simulink model "test_hill_sim"  (R2014b)
settings: Solver=ode113  StartTime=0.0  StopTime=t_end_CW  MaxStep=1e-3  MinStep=1e-12  RelTol=1e-9  AbsTol=1e-4
values from neighbouring files (symbols this model uses):
  a_sat = f_sat/m_cubesat    (= 0.0004)    [Controlled_motion_test1.m]    (also in Hill_TEST.m; TRAJ_Hill_test.m; controlled_motion_test2.m = 0.001)
  h_orb = 400*10^3    (= 400000)    [ATV_laplace_potentials_test0.m]    (also in CW_anlytical.m = 200000; Controlled_motion_test1.m; EOS_test.m = 250000; Hill_TEST.m = 800000)
  K_lqr = -K    [Controlled_motion_test1.m]    (also in Hill_TEST.m; TRAJ_Hill_test.m; controlled_motion_test2.m)
  Kp = kp    (= -0.075)    [Controlled_motion_test1.m]    (also in Hill_TEST.m = -7.5e-05; controlled_motion_test2.m; r2BP_t_c_CTR_SP.m = [kp 0 0)
  Kv = kv    (= -50)    [Controlled_motion_test1.m]    (also in Hill_TEST.m = -0.05; controlled_motion_test2.m; r2BP_t_c_CTR_SP.m = [kv 0 0)
  m_cubesat = 5    [Controlled_motion_test1.m]    (also in Hill_TEST.m; TRAJ_Hill_test.m; controlled_motion_test2.m)
  Mu = (3.9856e+14)    (= 398560000000000)    [ATV_laplace_potentials_test0.m]    (also in CW_anlytical.m; Controlled_motion_test1.m; EOS_test.m; Hill_TEST.m)
  R_0c = (R_0t+rand(3,1)*0.25*1e2)    [ATV_laplace_potentials_test0.m]    (also in CW_anlytical.m = [R_C;0;0]; Controlled_motion_test1.m = (R_0t+X_obs+rand(3,1)*0.25*1e2); Hill_TEST.m = (R_0t-rand(3,1)*0.5*1e2); Hill_TEST_INTEGR.m = (R_0t-[d_TC;0;0]))
  R_0t = [R_T;0;0]    [CW_anlytical.m]    (also in Controlled_motion_test1.m = [(r_Earth+h_orb);0;0]; EOS_test.m = [(r_Earth+h_orb);0;0]; Hill_TEST.m = [(r_Earth+h_orb);0;0]; Hill_TEST_INTEGR.m = [(r_Earth+h_orb);0;0])
  V_0c = (V_0t+rand(3,1)*0.5*1e-1)    [ATV_laplace_potentials_test0.m]    (also in CW_anlytical.m = [0;sqrt(Mu/norm(R_0c));0]; Controlled_motion_test1.m = (V_0t-rand(3,1)*0.25*1e-2); Hill_TEST.m; Hill_TEST_INTEGR.m = [0;omega*R_C;0])
  V_0t = [0;sqrt(Mu/(r_Earth+h_orb));0]    [CW_anlytical.m]    (also in Controlled_motion_test1.m; EOS_test.m; Hill_TEST.m; Hill_TEST_INTEGR.m)
undefined symbols (not defined in the file or in its folder): E, E_Moon, r_0, v_0
libraries: dspmtrx3 x4, vrlib x2
settings Model: Creator=peace  LastModifiedBy=peace

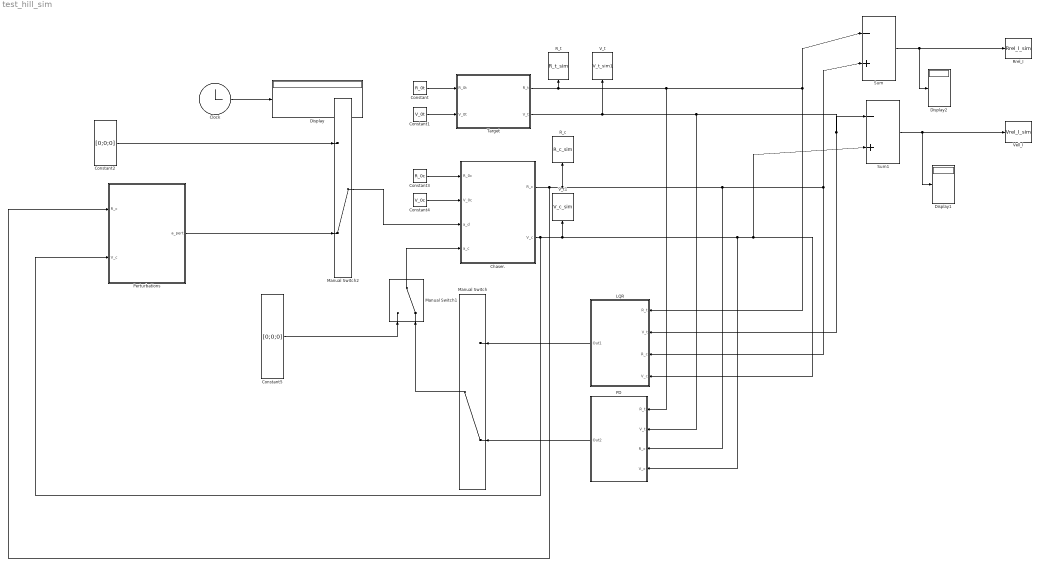
== system test_hill_sim ==
  Chaser. : Subsystem
  Clock : Clock
  Constant : Constant  Value=R_0t  VectorParams1D=off
  Constant1 : Constant  Value=V_0t  VectorParams1D=off
  Constant2 : Constant  Value=[0;0;0]  VectorParams1D=off
  Constant3 : Constant  Value=R_0c  VectorParams1D=off
  Constant4 : Constant  Value=V_0c  VectorParams1D=off
  Constant5 : Constant  Value=[0;0;0]  VectorParams1D=off
  Display : Display
  Display1 : Display
  Display2 : Display
  LQR : Subsystem
  Manual Switch : ManualSwitch  CurrentSetting=0
  Manual Switch1 : ManualSwitch  CurrentSetting=0
  Manual Switch2 : ManualSwitch  CurrentSetting=0
  PD : Subsystem
  Perturbations : Subsystem
  R_c : ToWorkspace  VariableName=R_c_sim  SaveFormat=Structure With Time  SampleTime=-1
  R_t : ToWorkspace  VariableName=R_t_sim  SaveFormat=Structure With Time  SampleTime=-1
  Rrel_I : ToWorkspace  VariableName=Rrel_I_sim  SaveFormat=Structure With Time  SampleTime=-1
  Sum : Sum  Inputs=|-+
  Sum1 : Sum  Inputs=|-+
  Target : Subsystem
  V_t : ToWorkspace  VariableName=V_t_sim1  SaveFormat=Structure With Time  SampleTime=-1
  V_t1 : ToWorkspace  VariableName=V_c_sim  SaveFormat=Structure With Time  SampleTime=-1
  Vell_I : ToWorkspace  VariableName=Vrel_I_sim  SaveFormat=Structure With Time  SampleTime=-1
  wires:
  Target/1(R_t) -> R_t/1, PD/1(R_t), LQR/1(R_t), Sum/1
  Constant/1 -> Target/1(R_0t)
  Constant1/1 -> Target/2(V_0t)
  Constant3/1 -> Chaser./1(R_0c)
  Constant4/1 -> Chaser./2(V_0c)
  Target/2("V_t ") -> V_t/1, PD/2(V_t), Sum1/1, LQR/2(V_t)
  Chaser./1(R_c) -> PD/3(R_c), LQR/3(R_c), Sum/2, R_c/1, Perturbations/1("R_c ")
  Chaser./2(V_c) -> Perturbations/2("V_c "), Sum1/2, LQR/4(V_c), PD/4(V_c), V_t1/1
  LQR/1(Out1) -> Manual Switch/1
  PD/1(Out2) -> Manual Switch/2
  Manual Switch1/1 -> Chaser./4(a_c)
  Constant5/1 -> Manual Switch1/1
  Manual Switch/1 -> Manual Switch1/2
  Perturbations/1(a_pert) -> Manual Switch2/2
  Manual Switch2/1 -> Chaser./3(a_d)
  Constant2/1 -> Manual Switch2/1
  Clock/1 -> Display/1
  Sum/1 -> Display2/1, Rrel_I/1
  Sum1/1 -> Display1/1, Vell_I/1

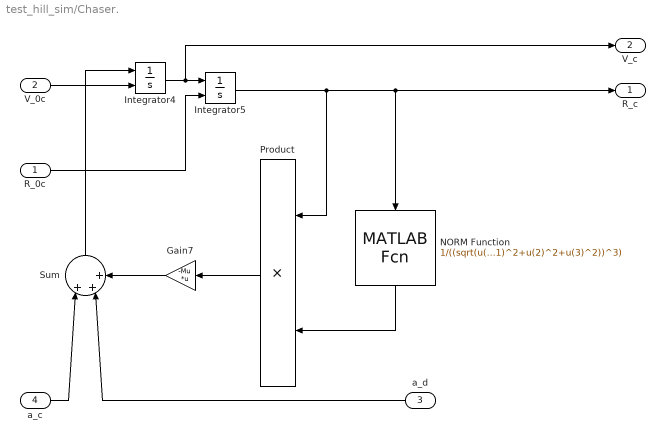
== system test_hill_sim/Chaser. ==
  R_0c : Inport
  V_0c : Inport  Port=2
  a_d : Inport  Port=3
  a_c : Inport  Port=4
  Gain7 : Gain  Gain=-Mu  Multiplication=Matrix(K*u)
  Integrator4 : Integrator  InitialConditionSource=external  InitialCondition=v_0
  Integrator5 : Integrator  InitialConditionSource=external  InitialCondition=r_0
  NORM Function : MATLABFcn  MATLABFcn=1/((sqrt(u(1)^2+u(2)^2+u(3)^2))^3)  OutputDimensions=1
  Product : Product
  Sum : Sum  Inputs=|+++
  R_c : Outport
  V_c : Outport  Port=2
  wires:
  Integrator5/1 -> R_c/1, NORM Function/1, Product/1
  Integrator4/1 -> Integrator5/1, V_c/1
  Product/1 -> Gain7/1
  NORM Function/1 -> Product/2
  V_0c/1 -> Integrator4/2
  R_0c/1 -> Integrator5/2
  Gain7/1 -> Sum/3
  Sum/1 -> Integrator4/1
  a_d/1 -> Sum/2
  a_c/1 -> Sum/1

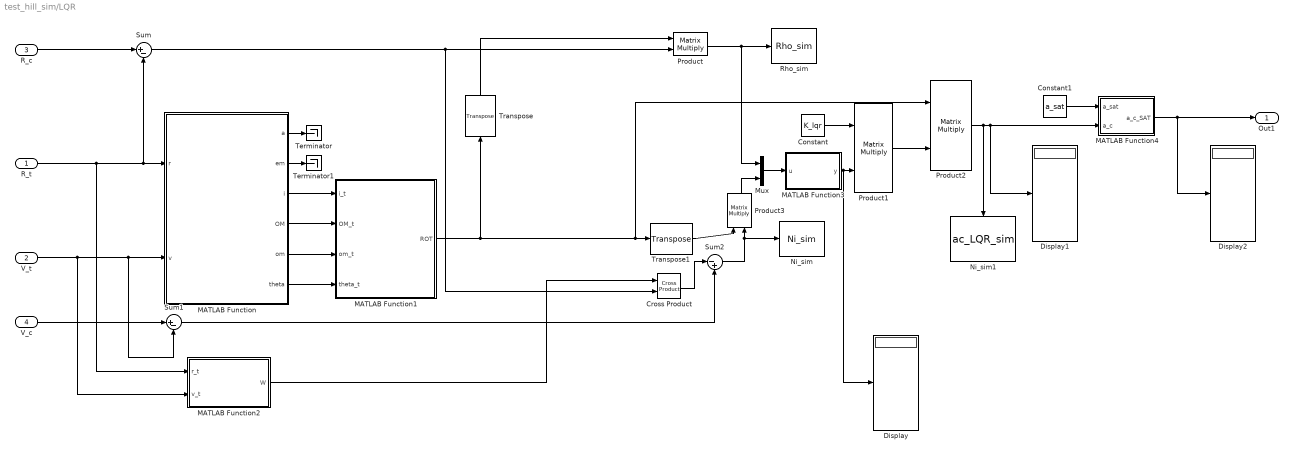
== system test_hill_sim/LQR ==
  R_t : Inport
  V_t : Inport  Port=2
  R_c : Inport  Port=3
  V_c : Inport  Port=4
  Constant : Constant  Value=K_lqr  VectorParams1D=off
  Constant1 : Constant  Value=a_sat
  Cross Product : vrlib/Utilities/Cross Product
  Display : Display
  Display1 : Display
  Display2 : Display
  MATLAB Function : MATLAB Function  TreatAsAtomicUnit=on
  MATLAB Function1 : MATLAB Function  TreatAsAtomicUnit=on
  MATLAB Function2 : MATLAB Function  TreatAsAtomicUnit=on
  MATLAB Function3 : MATLAB Function  TreatAsAtomicUnit=on
  MATLAB Function4 : MATLAB Function  TreatAsAtomicUnit=on
  Mux : Mux  Inputs=2
  Ni_sim : ToWorkspace  VariableName=Ni_sim  SaveFormat=Structure With Time  SampleTime=-1
  Ni_sim1 : ToWorkspace  VariableName=ac_LQR_sim  SaveFormat=Structure With Time  SampleTime=-1
  Product{,1..3} (4 alike) : Product  Multiplication=Matrix(*)
  Rho_sim : ToWorkspace  VariableName=Rho_sim  SaveFormat=Structure With Time  SampleTime=-1
  Sum : Sum  Inputs=|+-
  Sum1 : Sum  Inputs=|+-
  Sum2 : Sum  Inputs=|-+
  Terminator : Terminator
  Terminator1 : Terminator
  Transpose : dspmtrx3/Transpose  Hermitian=off  overflowFlag=off
  Transpose1 : dspmtrx3/Transpose  Hermitian=off  overflowFlag=off
  Out1 : Outport
  wires:
  R_t/1 -> Sum/2, MATLAB Function/1(r), MATLAB Function2/1(r_t)
  V_t/1 -> Sum1/2, MATLAB Function/2(v), MATLAB Function2/2(v_t)
  MATLAB Function/1(a) -> Terminator/1
  MATLAB Function/2(em) -> Terminator1/1
  MATLAB Function/3(i) -> MATLAB Function1/1(i_t)
  MATLAB Function/6(theta) -> MATLAB Function1/4(theta_t)
  MATLAB Function/4(OM) -> MATLAB Function1/2(OM_t)
  MATLAB Function/5(om) -> MATLAB Function1/3(om_t)
  R_c/1 -> Sum/1
  MATLAB Function1/1(ROT) -> Transpose/1, Product2/1, Transpose1/1
  V_c/1 -> Sum1/1
  Sum1/1 -> Sum2/2
  Sum/1 -> Product/2, Cross Product/2
  Cross Product/1 -> Sum2/1
  Product/1 -> Mux/1, Rho_sim/1
  Sum2/1 -> Product3/2, Ni_sim/1
  Constant/1 -> Product1/1
  Product2/1 -> MATLAB Function4/2(a_c), Display1/1, Ni_sim1/1
  Product1/1 -> Product2/2
  MATLAB Function2/1(W) -> Cross Product/1
  Transpose/1 -> Product/1
  Transpose1/1 -> Product3/1
  Product3/1 -> Mux/2
  Mux/1 -> MATLAB Function3/1(u)
  MATLAB Function3/1(y) -> Display/1, Product1/2
  MATLAB Function4/1(a_c_SAT) -> Display2/1, Out1/1
  Constant1/1 -> MATLAB Function4/1(a_sat)

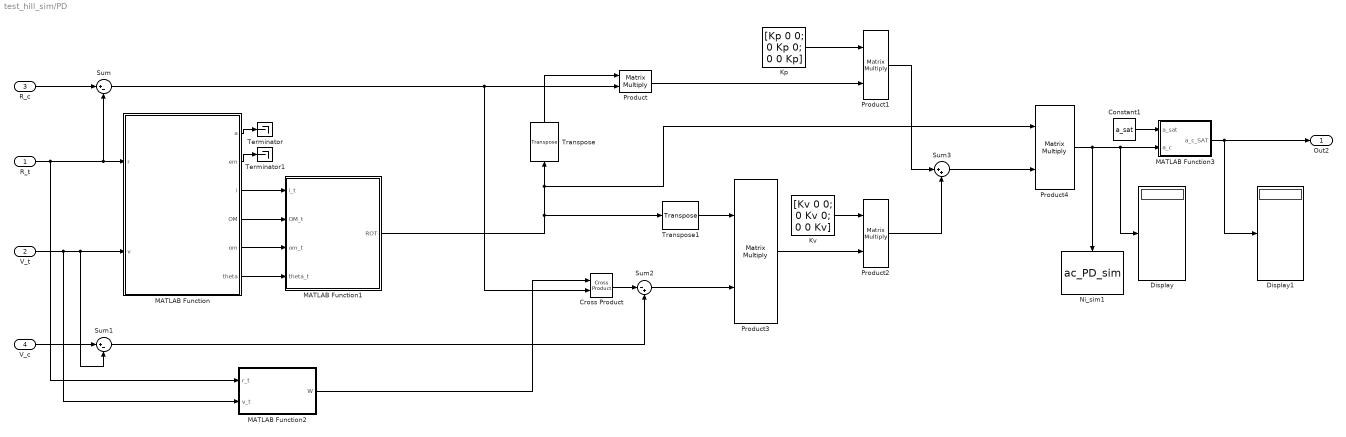
== system test_hill_sim/PD ==
  R_t : Inport
  V_t : Inport  Port=2
  R_c : Inport  Port=3
  V_c : Inport  Port=4
  Constant1 : Constant  Value=a_sat
  Cross Product : vrlib/Utilities/Cross Product
  Display : Display
  Display1 : Display
  Kp : Constant  Value=[Kp 0 0; 0 Kp 0; 0 0 Kp]  VectorParams1D=off
  Kv : Constant  Value=[Kv 0 0; 0 Kv 0; 0 0 Kv]  VectorParams1D=off
  MATLAB Function : MATLAB Function  TreatAsAtomicUnit=on
  MATLAB Function1 : MATLAB Function  TreatAsAtomicUnit=on
  MATLAB Function2 : MATLAB Function  TreatAsAtomicUnit=on
  MATLAB Function3 : MATLAB Function  TreatAsAtomicUnit=on
  Ni_sim1 : ToWorkspace  VariableName=ac_PD_sim  SaveFormat=Structure With Time  SampleTime=-1
  Product{,1..4} (5 alike) : Product  Multiplication=Matrix(*)
  Sum : Sum  Inputs=|+-
  Sum1 : Sum  Inputs=|+-
  Sum2 : Sum  Inputs=|-+
  Sum3 : Sum  Inputs=|++
  Terminator : Terminator
  Terminator1 : Terminator
  Transpose : dspmtrx3/Transpose  Hermitian=off  overflowFlag=off
  Transpose1 : dspmtrx3/Transpose  Hermitian=off  overflowFlag=off
  Out2 : Outport
  wires:
  R_t/1 -> MATLAB Function/1(r), Sum/2, MATLAB Function2/1(r_t)
  V_t/1 -> MATLAB Function2/2(v_t), MATLAB Function/2(v), Sum1/2
  MATLAB Function/1(a) -> Terminator/1
  MATLAB Function/2(em) -> Terminator1/1
  MATLAB Function/3(i) -> MATLAB Function1/1(i_t)
  MATLAB Function/6(theta) -> MATLAB Function1/4(theta_t)
  MATLAB Function/4(OM) -> MATLAB Function1/2(OM_t)
  MATLAB Function/5(om) -> MATLAB Function1/3(om_t)
  R_c/1 -> Sum/1
  MATLAB Function1/1(ROT) -> Product4/1, Transpose/1, Transpose1/1
  V_c/1 -> Sum1/1
  Sum1/1 -> Sum2/2
  Cross Product/1 -> Sum2/1
  Product/1 -> Product1/2
  Kp/1 -> Product1/1
  Kv/1 -> Product2/1
  Sum2/1 -> Product3/2
  Product3/1 -> Product2/2
  Product2/1 -> Sum3/2
  Product1/1 -> Sum3/1
  Product4/1 -> Ni_sim1/1, MATLAB Function3/2(a_c), Display/1
  Sum3/1 -> Product4/2
  Sum/1 -> Product/2, Cross Product/2
  Transpose/1 -> Product/1
  MATLAB Function2/1(W) -> Cross Product/1
  Transpose1/1 -> Product3/1
  Constant1/1 -> MATLAB Function3/1(a_sat)
  MATLAB Function3/1(a_c_SAT) -> Display1/1, Out2/1

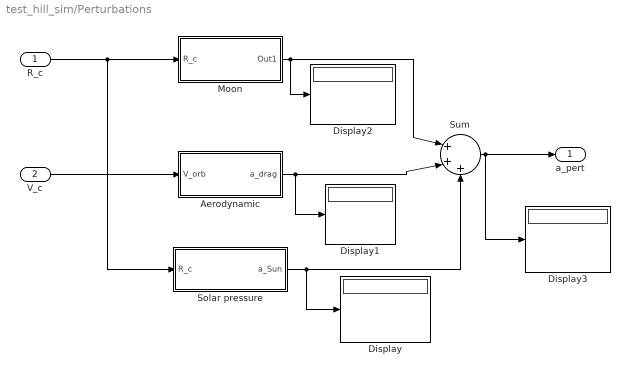
== system test_hill_sim/Perturbations ==
  "R_c " : Inport
  "V_c " : Inport  Port=2
  Aerodynamic : Subsystem
  Display{,1..3} (4 alike) : Display
  Moon : Subsystem
  Solar pressure : Subsystem
  Sum : Sum  Inputs=|+++
  a_pert : Outport
  wires:
  "R_c "/1 -> Solar pressure/1(R_c), Moon/1(R_c)
  Moon/1(Out1) -> Display2/1, Sum/1
  Sum/1 -> Display3/1, a_pert/1
  Aerodynamic/1(a_drag) -> Display1/1, Sum/2
  Solar pressure/1("a_Sun ") -> Display/1, Sum/3
  "V_c "/1 -> Aerodynamic/1(V_orb)

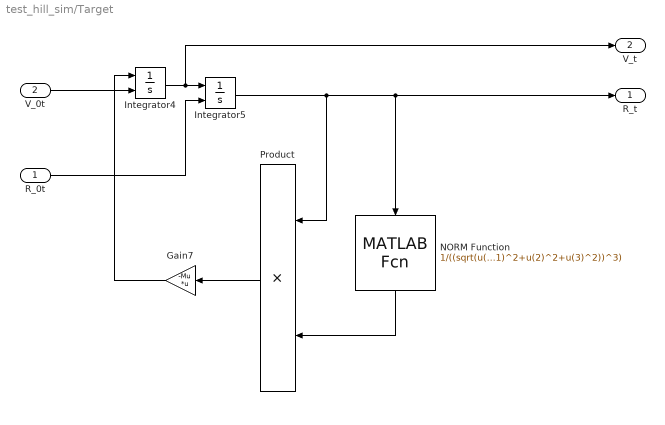
== system test_hill_sim/Target ==
  R_0t : Inport
  V_0t : Inport  Port=2
  Gain7 : Gain  Gain=-Mu  Multiplication=Matrix(K*u)
  Integrator4 : Integrator  InitialConditionSource=external  InitialCondition=v_0
  Integrator5 : Integrator  InitialConditionSource=external  InitialCondition=r_0
  NORM Function : MATLABFcn  MATLABFcn=1/((sqrt(u(1)^2+u(2)^2+u(3)^2))^3)  OutputDimensions=1
  Product : Product
  R_t : Outport
  "V_t " : Outport  Port=2
  wires:
  Integrator5/1 -> R_t/1, NORM Function/1, Product/1
  Integrator4/1 -> Integrator5/1, "V_t "/1
  Gain7/1 -> Integrator4/1
  Product/1 -> Gain7/1
  NORM Function/1 -> Product/2
  V_0t/1 -> Integrator4/2
  R_0t/1 -> Integrator5/2

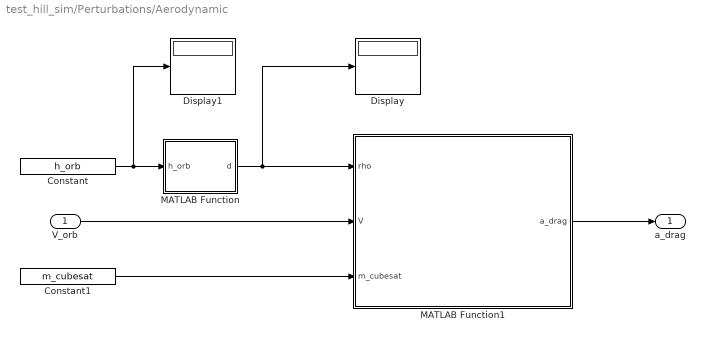
== system test_hill_sim/Perturbations/Aerodynamic ==
  V_orb : Inport
  Constant : Constant  Value=h_orb
  Constant1 : Constant  Value=m_cubesat
  Display : Display
  Display1 : Display
  MATLAB Function : MATLAB Function  TreatAsAtomicUnit=on
  MATLAB Function1 : MATLAB Function  TreatAsAtomicUnit=on
  a_drag : Outport
  wires:
  V_orb/1 -> MATLAB Function1/2(V)
  MATLAB Function1/1(a_drag) -> a_drag/1
  Constant/1 -> Display1/1, MATLAB Function/1(h_orb)
  MATLAB Function/1(d) -> Display/1, MATLAB Function1/1(rho)
  Constant1/1 -> MATLAB Function1/3(m_cubesat)

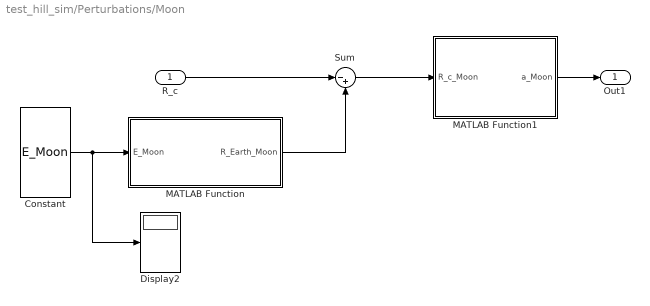
== system test_hill_sim/Perturbations/Moon ==
  R_c : Inport
  Constant : Constant  Value=E_Moon  VectorParams1D=off
  Display2 : Display
  MATLAB Function : MATLAB Function  TreatAsAtomicUnit=on
  MATLAB Function1 : MATLAB Function  TreatAsAtomicUnit=on
  Sum : Sum  Inputs=|-+
  Out1 : Outport
  wires:
  R_c/1 -> Sum/1
  MATLAB Function/1(R_Earth_Moon) -> Sum/2
  Sum/1 -> MATLAB Function1/1(R_c_Moon)
  MATLAB Function1/1(a_Moon) -> Out1/1
  Constant/1 -> Display2/1, MATLAB Function/1(E_Moon)

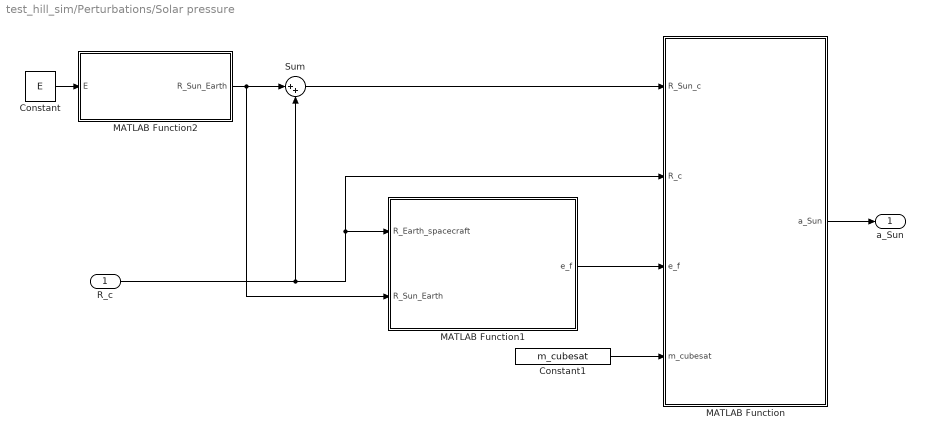
== system test_hill_sim/Perturbations/Solar pressure ==
  R_c : Inport
  Constant : Constant  Value=E  VectorParams1D=off
  Constant1 : Constant  Value=m_cubesat
  MATLAB Function : MATLAB Function  TreatAsAtomicUnit=on
  MATLAB Function1 : MATLAB Function  TreatAsAtomicUnit=on
  MATLAB Function2 : MATLAB Function  TreatAsAtomicUnit=on
  Sum : Sum  Inputs=|++
  "a_Sun " : Outport
  wires:
  R_c/1 -> Sum/2, MATLAB Function/2(R_c), MATLAB Function1/1(R_Earth_spacecraft)
  Sum/1 -> MATLAB Function/1(R_Sun_c)
  MATLAB Function1/1(e_f) -> MATLAB Function/3(e_f)
  MATLAB Function2/1(R_Sun_Earth) -> MATLAB Function1/2(R_Sun_Earth), Sum/1
  Constant/1 -> MATLAB Function2/1(E)
  Constant1/1 -> MATLAB Function/4(m_cubesat)
  MATLAB Function/1(a_Sun) -> "a_Sun "/1

== matlab function test_hill_sim/LQR/MATLAB Function1 ==
  data: i_t input; OM_t input; ROT output; om_t input; theta_t input
function ROT = PAR2ROT(i_t,OM_t,om_t,theta_t)
%#codegen

ROT=zeros(3,3);
ROT_plane=zeros(3,3);
ROT_theta=zeros(3,3);

ROT_plane=[cos(om_t)*cos(OM_t)-sin(om_t)*cos(i_t)*sin(OM_t) -sin(om_t)*cos(OM_t)-cos(om_t)*cos(i_t)*sin(OM_t) sin(i_t)*sin(OM_t)
    cos(om_t)*sin(OM_t)+sin(om_t)*cos(i_t)*cos(OM_t) -sin(om_t)*sin(OM_t)+cos(om_t)*cos(i_t)*cos(OM_t) -sin(i_t)*cos(OM_t)
    sin(om_t)*sin(i_t) cos(om_t)*sin(i_t) cos(i_t)]  ;

ROT_theta=[ cos(theta_t), sin(theta_t),0;
           -sin(theta_t), cos(theta_t),0;
                 0       ,    0       ,1];
             
            ROT=ROT_plane*ROT_theta;

end

== matlab function test_hill_sim/LQR/MATLAB Function ==
  data: r input; a output; v input; em output; i output; OM output; om output; theta output
function [a,em,i,OM,om,theta] = RV2ORBPAR(r,v)
%#codegen

mu=3.9856e+14;



v=[v(1);v(2);v(3)];
r=[r(1);r(2);r(3)];
rm=norm(r);
vm=norm(v);
a=mu/(((2*mu)/rm)-(vm^2));
h=cross(r,v);
hm=norm(h);
l=cross(v,h);
e=l/mu-r/rm;
em=norm(e);
i=acos(h(3)/hm);
kv=[0;0;1];
jv=[0;1;0];
iv=[1;0;0];

if norm(cross(kv,h))==0
n=iv;  
else
n=cross(kv,h)/norm(cross(kv,h));
end

    if dot(n,jv)>0
        OM=acos(dot(n,iv));
    else
        OM=2*pi-acos(dot(n,iv));
    end

if em==0
    
   om=0;
else
    
    if dot(e,kv)>0
        om=acos(dot(n,e)/em);
    else
        om=2*pi-acos(dot(n,e)/em);
    end
end

if em==0;

    theta=acos(dot(r/rm,iv));
    
else
     
   if em < 1e-7
    theta=acos(dot(r./rm,iv));
     
  else

    if dot(r,v)>0
        theta=acos(dot(r,e)/(rm*em));
    else
        theta=2*pi-acos(dot(r,e)/(rm*em));
    end
  end
end


end

== matlab function test_hill_sim/PD/MATLAB Function ==
  data: r input; a output; v input; em output; i output; OM output; om output; theta output
function [a,em,i,OM,om,theta] = RV2ORBPAR(r,v)
%#codegen

mu=3.9856e+14;



v=[v(1);v(2);v(3)];
r=[r(1);r(2);r(3)];
rm=norm(r);
vm=norm(v);
a=mu/(((2*mu)/rm)-(vm^2));
h=cross(r,v);
hm=norm(h);
l=cross(v,h);
e=l/mu-r/rm;
em=norm(e);
i=acos(h(3)/hm);
kv=[0;0;1];
jv=[0;1;0];
iv=[1;0;0];

if norm(cross(kv,h))==0
n=iv;  
else
n=cross(kv,h)/norm(cross(kv,h));
end

    if dot(n,jv)>0
        OM=acos(dot(n,iv));
    else
        OM=2*pi-acos(dot(n,iv));
    end

if em==0
    
   om=0;
else
    
    if dot(e,kv)>0
        om=acos(dot(n,e)/em);
    else
        om=2*pi-acos(dot(n,e)/em);
    end
end

if em==0;

    theta=acos(dot(r/rm,iv));
    
else
     
   if em < 1e-7
    theta=acos(dot(r./rm,iv));
     
  else

    if dot(r,v)>0
        theta=acos(dot(r,e)/(rm*em));
    else
        theta=2*pi-acos(dot(r,e)/(rm*em));
    end
  end
end


end

== matlab function test_hill_sim/PD/MATLAB Function1 ==
  data: i_t input; OM_t input; ROT output; om_t input; theta_t input
function ROT = PAR2ROT(i_t,OM_t,om_t,theta_t)
%#codegen
ROT=zeros(3,3);

ROT_plane=[cos(om_t)*cos(OM_t)-sin(om_t)*cos(i_t)*sin(OM_t) -sin(om_t)*cos(OM_t)-cos(om_t)*cos(i_t)*sin(OM_t) sin(i_t)*sin(OM_t)
    cos(om_t)*sin(OM_t)+sin(om_t)*cos(i_t)*cos(OM_t) -sin(om_t)*sin(OM_t)+cos(om_t)*cos(i_t)*cos(OM_t) -sin(i_t)*cos(OM_t)
    sin(om_t)*sin(i_t) cos(om_t)*sin(i_t) cos(i_t)]  ;

ROT_theta=[ cos(theta_t), sin(theta_t),0;
           -sin(theta_t), cos(theta_t),0;
                 0       ,    0       ,1];
             
            ROT=ROT_plane*ROT_theta;

end

== matlab function test_hill_sim/PD/MATLAB Function2 ==
  data: r_t input; W output; v_t input
function  W= w_gen(r_t,v_t)
%#codegen
v_t=[v_t(1);v_t(2);v_t(3)];
r_t=[r_t(1);r_t(2);r_t(3)];
W=zeros(3,1);
W=cross(r_t,v_t)/(norm(r_t)^2);
end

== matlab function test_hill_sim/LQR/MATLAB Function2 ==
  data: r_t input; W output; v_t input
function  W= w_gen(r_t,v_t)
%#codegen
v_t=[v_t(1);v_t(2);v_t(3)];
r_t=[r_t(1);r_t(2);r_t(3)];
W=zeros(3,1);
W=cross(r_t,v_t)/(norm(r_t)^2);
end

== matlab function test_hill_sim/Perturbations/Moon/MATLAB Function ==
  data: R_Earth_Moon output; E_Moon input
function R_Earth_Moon = Moon_Ef(E_Moon)
%#codegen
R_Earth_Moon=zeros(3,1);

E=E_Moon;
a=E(1)*1e3;
e=E(2);
i=E(3);
OM=E(4);
om=E(5);
theta=E(6);
i=i*pi/180;
OM=OM*pi/180;
om=om*pi/180;
theta=theta*pi/180;



r_pe=(a*(1-e^2))/(1+e*cos(theta));
r_PE=[r_pe*cos(theta) r_pe*sin(theta) 0]';
p=a*(1-e^2);





ROT=[cos(om)*cos(OM)-sin(om)*cos(i)*sin(OM) -sin(om)*cos(OM)-cos(om)*cos(i)*sin(OM) sin(i)*sin(OM)
    cos(om)*sin(OM)+sin(om)*cos(i)*cos(OM) -sin(om)*sin(OM)+cos(om)*cos(i)*cos(OM) -sin(i)*cos(OM)
    sin(om)*sin(i) cos(om)*sin(i) cos(i)];   
    
R_Earth_Moon=ROT*r_PE;

end

== matlab function test_hill_sim/Perturbations/Solar pressure/MATLAB Function ==
  data: R_Sun_c input; R_c input; e_f input; a_Sun output; m_cubesat input
function a_Sun=Sun_pert(R_Sun_c,R_c,e_f,m_cubesat)

%constants
a_Sun=zeros(3,1);

Power_Sun=1358; %[W/m^2]
Power_Earth_reflected=600;%[W/m^2](ALBEDO)
Power_Earth=150;%[W/m^2](IR)
c=299792458; %[m/s]
P_S=Power_Sun/c;
P_E=Power_Earth_reflected/c;
P_EE=Power_Earth/c;

%normalization of  condjungent vectors
S_s=R_Sun_c/norm(R_Sun_c);
S_e=R_c/norm(R_c);

%Panels data
a_p=0.3;%m
b_p=0.3;%m        
 
Ap=a_p*b_p;

%Ca_p = 0.80;
Cd_p = 0.10;
Cs_p = 0.10;

F_E=(e_f*P_E*Ap+P_EE*Ap)*S_e;
F_S=e_f*P_S*Ap*S_s;

a_Sun=F_S/m_cubesat+F_E/m_cubesat;
    




end

== matlab function test_hill_sim/Perturbations/Moon/MATLAB Function1 ==
  data: R_c_Moon input; a_Moon output
function a_Moon = Moon_pert(R_c_Moon)
%#codegen
a_Moon=zeros(3,1);
Mu_Earth=3.986e14;
Mu_Moon=0.012*Mu_Earth;
R_c_Moon_mod=norm(R_c_Moon);
a_Moon=-Mu_Moon/((R_c_Moon_mod)^3)*R_c_Moon;
end

== matlab function test_hill_sim/Perturbations/Solar pressure/MATLAB Function1 ==
  data: R_Earth_spacecraft input; R_Sun_Earth input; e_f output



function e_f =eclipse(R_Earth_spacecraft,R_Sun_Earth)

r_Earth=6378e3;

R_Earth_Sun=-R_Sun_Earth;

BETA=acos(dot(R_Earth_Sun,R_Earth_spacecraft)/(norm(R_Earth_Sun)*norm(R_Earth_spacecraft)));

if BETA>pi/2 && (norm(R_Earth_spacecraft)*sin(pi-BETA))<r_Earth
    e_f=0;
else
    e_f=1;
end

end

== matlab function test_hill_sim/Perturbations/Solar pressure/MATLAB Function2 ==
  data: R_Sun_Earth output; E input
function R_Sun_Earth = Earth_Ef(E)
%#codegen

R_Sun_Earth=zeros(3,1);

a=E(1)*1e3;
e=E(2);
i=E(3);
OM=E(4);
om=E(5);
theta=E(6);
i=i*pi/180;
OM=OM*pi/180;
om=om*pi/180;
theta=theta*pi/180;



r_pe=(a*(1-e^2))/(1+e*cos(theta));
r_PE=[r_pe*cos(theta) r_pe*sin(theta) 0]';






ROT=[cos(om)*cos(OM)-sin(om)*cos(i)*sin(OM) -sin(om)*cos(OM)-cos(om)*cos(i)*sin(OM) sin(i)*sin(OM)
    cos(om)*sin(OM)+sin(om)*cos(i)*cos(OM) -sin(om)*sin(OM)+cos(om)*cos(i)*cos(OM) -sin(i)*cos(OM)
    sin(om)*sin(i) cos(om)*sin(i) cos(i)];   
    
R_Sun_Earth=ROT*r_PE;
end

== matlab function test_hill_sim/Perturbations/Aerodynamic/MATLAB Function1 ==
  data: rho input; V input; a_drag output; m_cubesat input
function a_drag = pert_aero(rho,V,m_cubesat)
%#codegen



a_drag=zeros(3,1);
a_p=0.3;%m
b_p=0.3;%m        

Ap=a_p*b_p;

Cd_p=2; %(flat surface )


F_drag=-Ap*rho*(1/2)*Cd_p*norm(V)^2*(V/(norm(V)));

a_drag=F_drag/m_cubesat;
end

== matlab function test_hill_sim/Perturbations/Aerodynamic/MATLAB Function ==
  data: h_orb input; d output


function d  = spaceatm(h_orb)

h=h_orb/(1e3);

Z_km=[20    40    60    80   100   120   140   160   180   200   220   240   260   280   300   320   340   360   380   400 420   440   460   480   500   520   540   560   580   600   620   640   660   680   700   720   740   760   780   800 820   840   860   880];
d_km=[9.48E-02 4.07E-03 3.31E-04 1.69E-05 5.77E-07 1.70E-08 2.96E-09 9.65E-10 3.90E-10 1.75E-10 8.47E-11 4.31E-11 2.30E-11 1.27E-11 7.22E-12 4.21E-12 2.50E-12 1.51E-12 9.20E-13 5.68E-13 3.54E-13 2.23E-13 1.42E-13 9.20E-14 6.03E-14 4.03E-14 2.75E-14 1.93E-14 1.39E-14 1.03E-14 7.90E-15 6.24E-15 5.06E-15 4.21E-15 3.58E-15 3.09E-15 2.70E-15 2.39E-15 2.13E-15 1.91E-15 1.73E-15 1.56E-15 1.42E-15 1.30E-15];
[~,M]=size(Z_km);

h_top=0;
i_top=2;
for i=2:M
    h_test=Z_km(i);
    
    if h_test > h
        
        h_top= Z_km(i);
        i_top=i;
    end
    
   
end

d= d_km(i_top-1)+((d_km(i_top)-d_km(i_top-1))/(20))* (h-Z_km(i_top-1));
end

== matlab function test_hill_sim/LQR/MATLAB Function3 ==
  data: u input; y output
function y = correct_state_seq(u)
%#codegen
y=zeros(6,1);
y(1) = u(1);
y(2) = u(4);
y(3) = u(2);
y(4) = u(5);
y(5) = u(3);
y(6)=u(6);
end

== matlab function test_hill_sim/LQR/MATLAB Function4 ==
  data: a_sat input; a_c input; a_c_SAT output
function a_c_SAT = saturation(a_sat,a_c)
%#codegen
a_c_SAT=zeros(3,1);
for j=1:3
    
    if  a_c(j) >  a_sat 
        
        a_c_SAT(j)=a_sat;
   
    elseif  a_c(j) < -a_sat
        
        a_c_SAT(j)=-a_sat;
    else
        a_c_SAT(j)=a_c(j);
    end
    
end

== matlab function test_hill_sim/PD/MATLAB Function3 ==
  data: a_sat input; a_c input; a_c_SAT output
function a_c_SAT = saturation(a_sat,a_c)
%#codegen
a_c_SAT=zeros(3,1);
for j=1:3
    
    if  a_c(j) >  a_sat 
        
        a_c_SAT(j)=a_sat;
   
    elseif  a_c(j) < -a_sat
        
        a_c_SAT(j)=-a_sat;
    else
        a_c_SAT(j)=a_c(j);
    end
    
end
